simulink model "Integration"  (R2024b)
settings: Solver=VariableStepAuto  StartTime=0.0  StopTime=10.0  RelTol=1e-3
undefined symbols (not defined in the file): lambda
libraries: robotmaniplib x5, robotcorelib x3, slpidlib x1, dspinverses x1, robotsim3dlib x1, sim3dlib x1
settings Model: Creator=kiwiki  LastModifiedBy=dd217

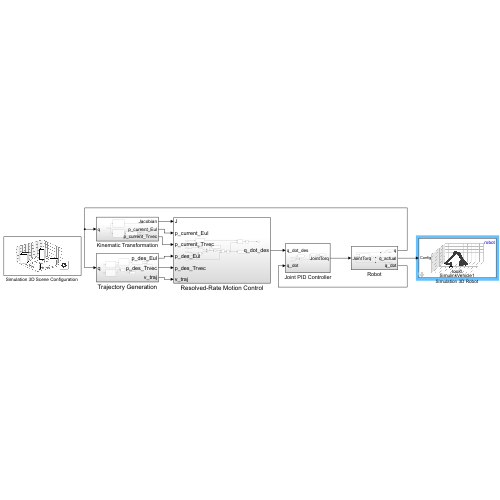
[thumbnail: Simulink's stored preview of the top-level diagram]
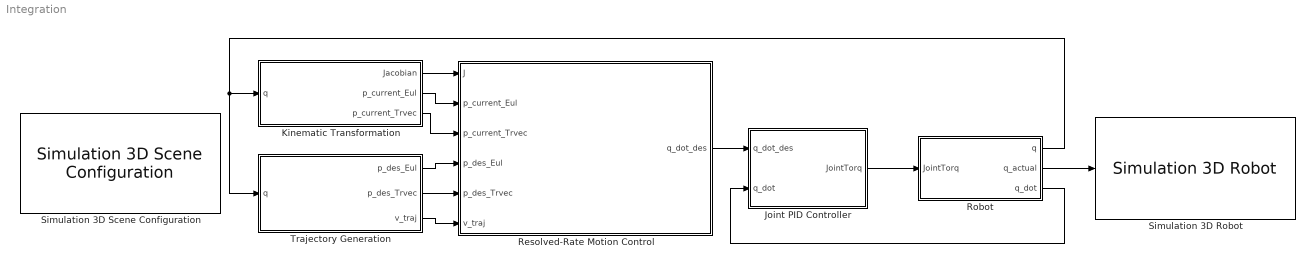
== system Integration ==
  Joint PID Controller : Subsystem
  Kinematic Transformation : Subsystem
  Resolved-Rate Motion Control : Subsystem
  Robot : Subsystem
  "Simulation 3D Robot " : robotsim3dlib/Simulation 3D Robot  actorInputType=RigidBodyTree Object  RigidBodyTree=robot  ActorName=SimulinkVehicle1  existActorChekBox=off  initialTrans=[0 0 0]  initialRot=[0 0 0]  initialConfig=[0 0 0 0 0 0]  EndEffector=tool0  eeOffsetInpChekBox=off  eeTargetTrans=[0 0 0]  eeTargetRot=[0 0 0]  enableRegionGraspChekBox=off  regionGraspInpChekBox=off  eeTargTransDiff=[0.2 0.2 0.2]  eeTargRotDiff=[0 0 0]  inpConfEnbVal=on  inpGraspEnbVal=off  inpTransEnbVal=off  outConfEnbVal=off  outGraspEnbVal=off  outTransEnbVal=off  SampleTime=0.01  ActorType=SimulinkVehicle  ID=1  aMode=6  ActorTag=SimulinkVehicle1  Mesh=RigidBodyTree
  "Simulation 3D Scene Configuration " : sim3dlib/Simulation 3D Scene Configuration  Priority=0  ProjectFormat=Default Scenes  SceneDesc=Empty scene  ProjectName=C:\Program Files\MATLAB\R2024b\toolbox\shared\sim3d_projects\automotive_project_windows\UE\WindowsNoEditor\VehicleSimulation.exe  ScenePath=/Game/Maps/EmptyScene  EnableOpenDRIVE=off  vehTagList={'Custom';'Scene Origin';'SimulinkVehicle1'}  vehTag=Scene Origin  FreeCameraInitialTranslation=[0, 0, 0]  FreeCameraDefaultInitialTranslation=[-6, 0, 2]  FreeCameraInitialRotation=[0, 0, 0]  FreeCameraDefaultInitialRotation=[0, -15, 0]  OpVisEn=off  Ts=0.01  EnableWindow=on  EnableRemoteAccess=off  EnableWeather=off  SunAzimuth=90  SunAltitude=40.0  EnableGeospatialSun=off  Latitude=0  Longitude=0  Date=2023-01-01  Time=10:30:00  GeoTimeZone=-5.0  SunDaylightSaving=off  wind=1  clouds=10  EnableVolumetricClouds=off  CloudCoverage=0  CloudAltitude=6  fog=0  rain=0  RaindropsEffect=off  SnowDensity=0  EnableGeospatial=off  UseTrueOrigin=off  OriginHeight=200  OriginLatitude=40.744652  OriginLongitude=-73.988864  MapStyle=Aerial  AdditionalAssetIDs=[]  UseAdvancedSunSky=off  SolarTime=11  TimeZone=-5  Day=21  Month=9  Year=2022  UseDaylightSavingTime=on  DSTStartDay=10  DSTStartMonth=3  DSTEndDay=3  DSTEndMonth=11  DSTSwitchHour=2  sensorTag=MainCamera1  sensorId=1  sensorName=MainCamera1  mountLoc=Origin  offsetFlag=off  tmountOffset=[0, 0, 0]  rmountOffset=[0, 0, 0]  HorizontalResolution=1280  VerticalResolution=720  HorizontalFOV=60  mountPoint=[0 0 0]  mountOrientation=[0 0 0]  aMode=6  ID=1  GeoTrigger=Inactive
      settings: LibrarySourceBlock=robotsim3dlib/Simulation 3D Scene Configuration
  Trajectory Generation : Subsystem
  wires:
  Kinematic Transformation/1(Jacobian) -> Resolved-Rate Motion Control/1(J)
  Kinematic Transformation/2(p_current_Eul) -> Resolved-Rate Motion Control/2(p_current_Eul)
  Kinematic Transformation/3(p_current_Trvec) -> Resolved-Rate Motion Control/3(p_current_Trvec)
  Trajectory Generation/1(p_des_Eul) -> Resolved-Rate Motion Control/4(p_des_Eul)
  Trajectory Generation/3(v_traj) -> Resolved-Rate Motion Control/6(v_traj)
  Trajectory Generation/2(p_des_Trvec) -> Resolved-Rate Motion Control/5(p_des_Trvec)
  Resolved-Rate Motion Control/1(q_dot_des) -> Joint PID Controller/1(q_dot_des)
  Robot/1(q) -> Trajectory Generation/1(q), Kinematic Transformation/1(q)
  Joint PID Controller/1(JointTorq) -> Robot/1(JointTorq)
  Robot/3(q_dot) -> Joint PID Controller/2(q_dot)
  Robot/2(q_actual) -> "Simulation 3D Robot "/1

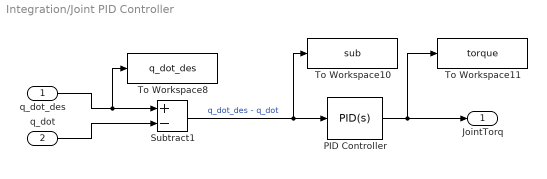
== system Integration/Joint PID Controller ==
  q_dot_des : Inport
  q_dot : Inport  Port=2
  "PID Controller " : slpidlib/PID Controller  Controller=PID  Form=Parallel  TimeDomain=Continuous-time  UseExternalTs=off  SampleTime=-1  IntegratorMethod=Forward Euler  FilterMethod=Forward Euler  ControllerParametersSource=internal  P=7.5  I=0.01  UseKiTs=off  D=1.3  UseExternalDerivativeSource=off  N=60  UseFilter=on  TunerSelectOption=Transfer Function Based (PID Tuner App)  InitialConditionSource=internal  InitialConditionForIntegrator=0  InitialConditionForFilter=0  DifferentiatorICPrevScaledInput=0  ExternalReset=none  TrackingMode=off  Kt=1  LimitOutput=on  SatLimitsSource=internal  UpperSaturationLimit=50  LowerSaturationLimit=-50  LinearizeAsGain=on  AntiWindupMode=back-calculation  Kb=1  LimitIntegrator=off  UpperIntegratorSaturationLimit=inf  LowerIntegratorSaturationLimit=-inf  POutMin=[]  POutMax=[]  IOutMin=[]  IOutMax=[]  DOutMin=[]  DOutMax=[]  NOutMin=[]  NOutMax=[]  SumOutMin=[]  SumOutMax=[]  SaturationOutMin=[]  SaturationOutMax=[]  PParamMin=[]  PParamMax=[]  IParamMin=[]  IParamMax=[]  DParamMin=[]  DParamMax=[]  NParamMin=[]  NParamMax=[]  KbParamMin=[]  KbParamMax=[]  KtParamMin=[]  KtParamMax=[]  KbOutMin=[]  KbOutMax=[]  KtOutMin=[]  KtOutMax=[]  IntegratorOutMin=[]  IntegratorOutMax=[]  FilterOutMin=[]  FilterOutMax=[]  SumI1OutMin=[]  SumI1OutMax=[]  SumI2OutMin=[]  SumI2OutMax=[]  SumI3OutMin=[]  SumI3OutMax=[]  SumI4OutMin=[]  SumI4OutMax=[]  SumDOutMin=[]  SumDOutMax=[]  DifferentiatorOutMin=[]  DifferentiatorOutMax=[]  FilterDiffOutCoefMin=[]  FilterDiffOutCoefMax=[]  ReciprocalOutMin=[]  ReciprocalOutMax=[]  SumDenOutMin=[]  SumDenOutMax=[]  SumNumOutMin=[]  SumNumOutMax=[]  DivideOutMin=[]  DivideOutMax=[]  UdiffTsProdOutMin=[]  UdiffTsProdOutMax=[]  NTsProdOutMin=[]  NTsProdOutMax=[]  UintegralTsProdOutMin=[]  UintegralTsProdOutMax=[]  UngainTsProdOutMin=[]  UngainTsProdOutMax=[]  ClampingZeroOutDataTypeStr=Inherit: Inherit via back propagation  ClampingZeroOutMin=[]  ClampingZeroOutMax=[]  FilterDenConstantOutDataTypeStr=Inherit: Inherit via back propagation  FilterDenConstantOutMin=[]  FilterDenConstantOutMax=[]  PCopyOutDataTypeStr=Inherit: Inherit via back propagation  PCopyOutMin=[]  PCopyOutMax=[]  NCopyOutDataTypeStr=Inherit: Inherit via back propagation  NCopyOutMin=[]  NCopyOutMax=[]  IntegratorContinuousStateAttributes=''  IntegratorStateMustResolveToSignalObject=off  IntegratorRTWStateStorageClass=Auto  FilterContinuousStateAttributes=''  FilterStateMustResolveToSignalObject=off  FilterRTWStateStorageClass=Auto  ParallelPVariant=InternalParameters  IdealPVariant=Disabled  IVariant=InternalParameters  DVariant=InternalParameters  IntegratorVariant=Continuous  SatVariant=Enabled  AWVariant=BackCalculation  PCopyVariant=Disabled  TRVariant=Disabled  FdbkBlocksVariant=Forward  IdealPFdbkVariant=Disabled  SatFdbkVariant=Disabled  DerivativeFilterVariant=ContFilter  NVariant=InternalParameters  NCopyVariant=Disabled  FilterICVariant=InternalICsFilter  IntegratorICVariant=InternalICs  ExternalResetVariant=Disabled  TRSumVariant=Passthrough  SumFdbkVariant=Disabled  SumVariant=Sum_PID  TsampFilterVariant=InternalTs  TsampNgainVariant=Passthrough  TsampIntegralVariant=Disabled_SignalSpec  ExternalSaturationOutDataTypeStr=Inherit: Same as second input  DerivativeSourceVariant=ErrorSignal  PreIntVariant=InternalPreInt
  Subtract1 : Sum  Inputs=+-
  To Workspace10 : ToWorkspace  VariableName=sub  SaveFormat=Structure With Time  SampleTime=0.01
  To Workspace11 : ToWorkspace  VariableName=torque  SaveFormat=Structure With Time  SampleTime=0.01
  To Workspace8 : ToWorkspace  VariableName=q_dot_des  SaveFormat=Structure With Time  SampleTime=0.01
  JointTorq : Outport
  wires:
  q_dot/1 -> Subtract1/2
  q_dot_des/1 -> To Workspace8/1, Subtract1/1
  Subtract1/1 -> "PID Controller "/1, To Workspace10/1  "q_dot_des - q_dot"
  "PID Controller "/1 -> To Workspace11/1, JointTorq/1

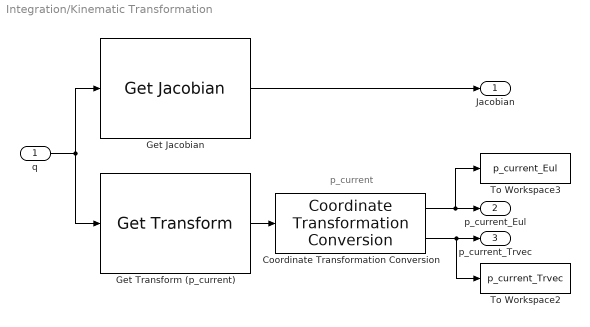
== system Integration/Kinematic Transformation ==
  note: p_current
  q : Inport
  Coordinate Transformation Conversion : robotcorelib/Coordinate Transformation Conversion  InputRepresentation=Homogeneous Transformation  InputEulerSequence=ZYX  ShowTrVecInputPort=on  OutputRepresentation=Euler Angles  OutputEulerSequence=ZYX  ShowTrVecOutputPort=on  SimulateUsing=Interpreted execution
  "Get Jacobian " : robotmaniplib/Get Jacobian  RigidBodyTree=robot  EndEffector=tool0  SimulateUsing=Interpreted execution
  Get Transform (p_current) : robotmaniplib/Get Transform  RigidBodyTree=robot  SourceBody=base_link  TargetBody=tool0  SimulateUsing=Interpreted execution
  To Workspace2 : ToWorkspace  VariableName=p_current_Trvec  SaveFormat=Structure With Time  SampleTime=0.01
  To Workspace3 : ToWorkspace  VariableName=p_current_Eul  SaveFormat=Structure With Time  SampleTime=0.01
  Jacobian : Outport
  p_current_Eul : Outport  Port=2
  p_current_Trvec : Outport  Port=3
  wires:
  "Get Jacobian "/1 -> Jacobian/1
  Get Transform (p_current)/1 -> Coordinate Transformation Conversion/1
  q/1 -> "Get Jacobian "/1, Get Transform (p_current)/1
  Coordinate Transformation Conversion/1 -> To Workspace3/1, p_current_Eul/1
  Coordinate Transformation Conversion/2 -> To Workspace2/1, p_current_Trvec/1

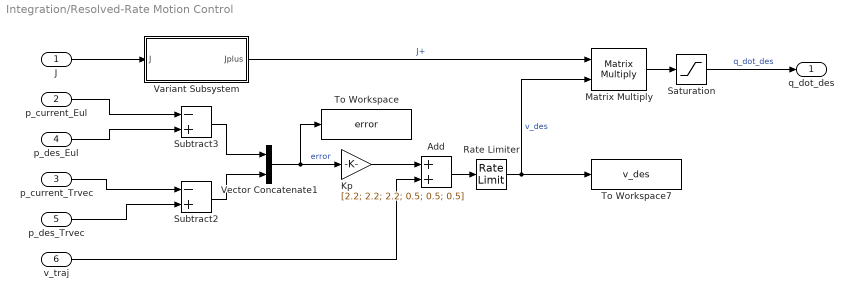
== system Integration/Resolved-Rate Motion Control ==
  J : Inport
  p_current_Eul : Inport  Port=2
  p_current_Trvec : Inport  Port=3
  p_des_Eul : Inport  Port=4
  p_des_Trvec : Inport  Port=5
  v_traj : Inport  Port=6
  Add : Sum
  Kp : Gain  Gain=[2.2; 2.2; 2.2; 0.5; 0.5; 0.5]
  Matrix Multiply : Product  Multiplication=Matrix(*)
  "Rate Limiter " : RateLimiter  RisingSlewLimit=[0.3; 0.3; 0.3; 0.8; 0.8; 0.8]  FallingSlewLimit=[-0.3; -0.3; -0.3; -0.8; -0.8; -0.8]  SampleTimeMode=inherited
  "Saturation " : Saturate  UpperLimit=1.6  LowerLimit=-1.6
  Subtract2 : Sum  Inputs=-+
  Subtract3 : Sum  Inputs=-+
  To Workspace : ToWorkspace  VariableName=error  SaveFormat=Structure With Time  SampleTime=0.01
  To Workspace7 : ToWorkspace  VariableName=v_des  SaveFormat=Structure With Time  SampleTime=0.01
  "Variant Subsystem " : Subsystem  Variant=on
  Vector Concatenate1 : Concatenate
  q_dot_des : Outport
  wires:
  v_traj/1 -> Add/2
  "Saturation "/1 -> q_dot_des/1  "q_dot_des"
  "Variant Subsystem "/1(Jplus) -> Matrix Multiply/1  "J+"
  Matrix Multiply/1 -> "Saturation "/1
  J/1 -> "Variant Subsystem "/1(J)
  Vector Concatenate1/1 -> To Workspace/1, Kp/1  "error"
  p_des_Trvec/1 -> Subtract2/2
  "Rate Limiter "/1 -> Matrix Multiply/2, To Workspace7/1  "v_des"
  Subtract2/1 -> Vector Concatenate1/2
  p_current_Trvec/1 -> Subtract2/1
  p_current_Eul/1 -> Subtract3/1
  p_des_Eul/1 -> Subtract3/2
  Subtract3/1 -> Vector Concatenate1/1
  Kp/1 -> Add/1
  Add/1 -> "Rate Limiter "/1

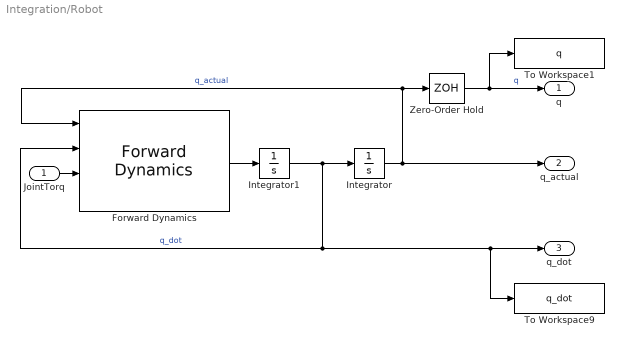
== system Integration/Robot ==
  JointTorq : Inport
  "Forward Dynamics " : robotmaniplib/Forward Dynamics  RigidBodyTree=robot  SimulateUsing=Interpreted execution
  "Integrator " : Integrator  InitialCondition=[0;0;0;0;0;0]
  "Integrator1 " : Integrator  InitialCondition=[0;0;0;0;0;0]
  To Workspace1 : ToWorkspace  VariableName=q  SaveFormat=Structure With Time  SampleTime=0.01
  To Workspace9 : ToWorkspace  VariableName=q_dot  SaveFormat=Structure With Time  SampleTime=0.01
  "Zero-Order Hold " : ZeroOrderHold  SampleTime=0.01
  q : Outport
  q_actual : Outport  Port=2
  q_dot : Outport  Port=3
  wires:
  "Integrator "/1 -> q_actual/1, "Forward Dynamics "/1, "Zero-Order Hold "/1  "q_actual"
  "Integrator1 "/1 -> "Forward Dynamics "/2, To Workspace9/1, q_dot/1, "Integrator "/1  "q_dot"
  "Forward Dynamics "/1 -> "Integrator1 "/1
  JointTorq/1 -> "Forward Dynamics "/3
  "Zero-Order Hold "/1 -> q/1, To Workspace1/1  "q"

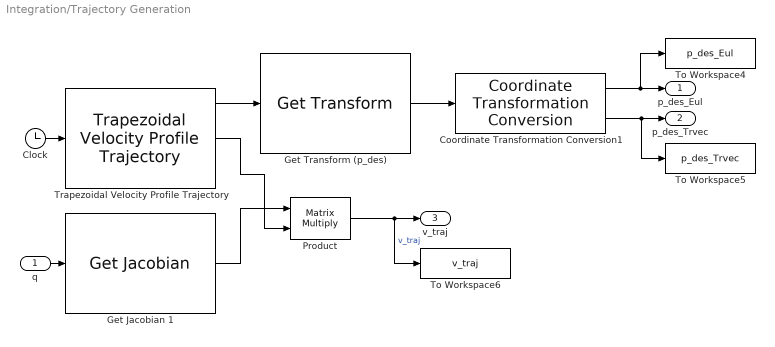
== system Integration/Trajectory Generation ==
  q : Inport
  "Clock " : Clock
  Coordinate Transformation Conversion1 : robotcorelib/Coordinate Transformation Conversion  InputRepresentation=Homogeneous Transformation  InputEulerSequence=ZYX  ShowTrVecInputPort=on  OutputRepresentation=Euler Angles  OutputEulerSequence=ZYX  ShowTrVecOutputPort=on  SimulateUsing=Interpreted execution
  Get Jacobian 1 : robotmaniplib/Get Jacobian  RigidBodyTree=robot  EndEffector=tool0  SimulateUsing=Interpreted execution
  Get Transform (p_des) : robotmaniplib/Get Transform  RigidBodyTree=robot  SourceBody=base_link  TargetBody=tool0  SimulateUsing=Interpreted execution
  Product : Product  Multiplication=Matrix(*)
  To Workspace4 : ToWorkspace  VariableName=p_des_Eul  SaveFormat=Structure With Time  SampleTime=0.01
  To Workspace5 : ToWorkspace  VariableName=p_des_Trvec  SaveFormat=Structure With Time  SampleTime=0.01
  To Workspace6 : ToWorkspace  VariableName=v_traj  SaveFormat=Structure With Time  SampleTime=0.01
  Trapezoidal Velocity Profile Trajectory : robotcorelib/Trapezoidal Velocity Profile Trajectory  WaypointSource=Internal  Waypoints=|  NumParams=2  Parameter1=Peak Velocity  Parameter2=Acceleration  ParameterSource=Internal  PeakVelocity=[0.05; 0.05; 0.05; 0.05; 0.05; 0.05]  Acceleration=[0.08; 0.08; 0.08; 0.08; 0.08; 0.08]  EndTime=[ 1; 1 ]  AccelTime=[ 1; 2 ]  SimulateUsing=Interpreted execution
      | [ 0   0.2   0.4   0.6;
      |   0   0     0     0;
      |   0   0     0     0;
      |   0   0     0     0;
      |   0   0     0     0;
      |   0   0     0     0 ]
  p_des_Eul : Outport
  p_des_Trvec : Outport  Port=2
  v_traj : Outport  Port=3
  wires:
  q/1 -> Get Jacobian 1/1
  Trapezoidal Velocity Profile Trajectory/2 -> Product/2
  Get Jacobian 1/1 -> Product/1
  Trapezoidal Velocity Profile Trajectory/1 -> Get Transform (p_des)/1
  "Clock "/1 -> Trapezoidal Velocity Profile Trajectory/1
  Get Transform (p_des)/1 -> Coordinate Transformation Conversion1/1
  Product/1 -> To Workspace6/1, v_traj/1  "v_traj"
  Coordinate Transformation Conversion1/1 -> To Workspace4/1, p_des_Eul/1
  Coordinate Transformation Conversion1/2 -> p_des_Trvec/1, To Workspace5/1

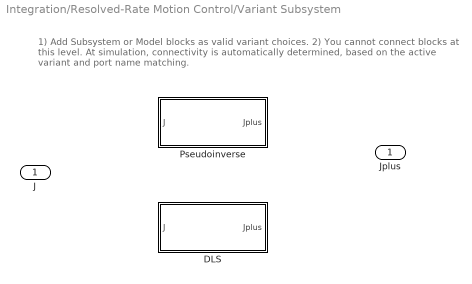
== system Integration/Resolved-Rate Motion Control/Variant Subsystem  ==
  note: 1) Add Subsystem or Model blocks as valid variant choices.
      | 2) You cannot connect blocks at this level. At simulation, connectivity is automatically
      | determined, based on the active variant and port name matching.
  J : Inport
  DLS : Subsystem  VariantControl=select==1
  Pseudoinverse : Subsystem  VariantControl=select==0
  Jplus : Outport

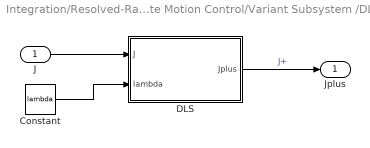
== system Integration/Resolved-Rate Motion Control/Variant Subsystem /DLS ==
  J : Inport
  " DLS" : MATLAB Function  TreatAsAtomicUnit=on
  Constant : Constant  Value=lambda
  Jplus : Outport
  wires:
  J/1 -> " DLS"/1(J)
  " DLS"/1(Jplus) -> Jplus/1  "J+"
  Constant/1 -> " DLS"/2(lambda)

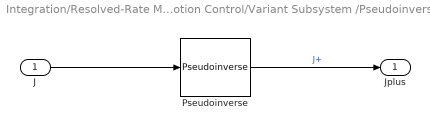
== system Integration/Resolved-Rate Motion Control/Variant Subsystem /Pseudoinverse ==
  J : Inport
  Pseudoinverse : dspinverses/Pseudoinverse  wanterr=off  SimulateUsing=Interpreted execution
  Jplus : Outport
  wires:
  J/1 -> Pseudoinverse/1
  Pseudoinverse/1 -> Jplus/1  "J+"

== matlab function Integration/Resolved-Rate Motion Control/Variant Subsystem /DLS/ DLS ==
  data: J input; Jplus output; lambda input
function Jplus = dls_pinv(J, lambda)
    % Damped Least Squares Pseudoinverse
    [m, n] = size(J);
    Jplus = J' / (J*J' + lambda^2*eye(m));
end
